simulink model "test_lookup_node"  (Simulink 7.7)
settings: Solver=FixedStepDiscrete  StartTime=0.0  StopTime=10000.0  FixedStep=1  RelTol=1e-3
libraries: LookupModeling x1
settings Model: Creator=medcps  LastModifiedBy=iris
settings DataIOCC: SignalLogging=off
settings OptimizationCC: BlockReduction=off  ConditionallyExecuteInputs=off  InlineParams=on
settings DebuggingCC: AlgebraicLoopMsg=error  FcnCallInpInsideContextMsg=Enable All
settings HardwareCC: ProdHWDeviceType=ASIC/FPGA->ASIC/FPGA

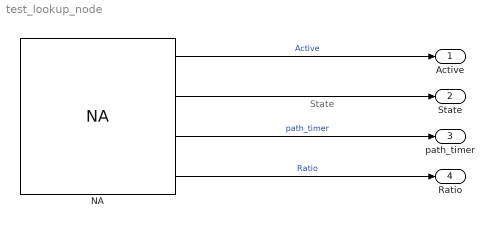
== system test_lookup_node ==
  note: State
  NA : LookupModeling/NA  SystemSampleTime=-1  TERP_s_m=320  TERP_defs_m=320  TRRP_s_m=100  TRRP_def_m=100  Trest_s_m=800  Trest_def_m=800  Terp_min_m=150  Terp_max_m=300
  Active : Outport
  State : Outport  Port=2
  path_timer : Outport  Port=3
  Ratio : Outport  Port=4
  wires:
  NA/1 -> Active/1  "Active"
  NA/2 -> State/1
  NA/3 -> path_timer/1  "path_timer"
  NA/4 -> Ratio/1  "Ratio"
